simulink model "oscillator"  (R2021a)
settings: Solver=FixedStepAuto  StartTime=0.0  StopTime=timeFinal  FixedStep=timeStepMax  MaxStep=timeStepMax  RelTol=1e-3
model workspace (MAT data in the model file):
  x0 = 5
  y0 = 5
values from neighbouring files (symbols this model uses):
  a = x0_0    [run_oscillator.m]
  b = x1_0    [run_oscillator.m]
settings Model: SimulationMode=accelerator  Creator=amit  LastModifiedBy=amit
settings DataIOCC: ExternalInput=[x0, y0]

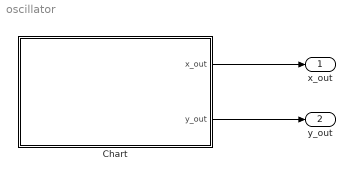
== system oscillator ==
  Chart : Stateflow chart  TreatAsAtomicUnit=on
  x_out : Outport  SignalName=xOut
  y_out : Outport  Port=2  SignalName=yOut
  wires:
  Chart/1(x_out) -> x_out/1
  Chart/2(y_out) -> y_out/1

== stateflow chart oscillator/Chart ==
  settings: updateMethod=CONTINUOUS  executeAtInitialization=1
  state loc4
    du:
    % derivatives
    % make x, y as continuous
    x_dot = -2.0 * x + 1.4;
    y_dot = -1.0 * y - 0.7;
    exit:
    x_out=x;
    y_out=y;
  state loc3
    du:
    % derivatives
    x_dot = -2.0 * x - 1.4;
    y_dot = -1.0 * y + 0.7;
    exit:
    x_out=x;
    y_out=y;
  state loc1
    du:
    % derivatives
    x_dot = -2.0 * x + 1.4;
    y_dot = -1.0 * y - 0.7;
    exit:
    x_out=x;
    y_out=y;
  state loc2
    du:
    x_dot = -2.0 * x - 1.4;
    y_dot = -1.0 * y + 0.7;
    exit:
    x_out=x;
    y_out=y;
  loc3 -> loc4 [order 1] : [y>=-0.714286 * x & x<=0]{x=x; y=y;}
  loc3 -> loc3 [order 2] : [y<-0.714286 * x & x<0]{x=x; y=y;}
  loc2 -> loc3 [order 2] : [y<-0.714286 * x & x<=0]{x=x; y=y;}
  loc4 -> loc1 [order 2] : [x>0 &  y >= -0.714286 * x] {x=x; y=y;}
  loc4 -> loc4 [order 1] : [y>-0.714286 * x & x<=0]{x=x; y=y;}
  loc1 -> loc1 [order 1] : [y>=-0.714286 * x & x>0]{x=x; y=y;}
  loc2 -> loc2 [order 1] : [y<-0.714286 * x & x>0]{x=x; y=y;}
  loc1 -> loc2 [order 2] : [y<-0.714286 * x & x>=0]{x=x; y=y;}
  (default) -> loc1 : {x=a; y=b;}
  data: x_out output; y_out output; y local; x local; a parameter; b parameter
  data y settings: updateMethod=SF_CONTINUOUS_TIME_DATA
  data x settings: updateMethod=SF_CONTINUOUS_TIME_DATA
